simulink model "cic"  (Simulink 7.1)
settings: Solver=FixedStepDiscrete  StartTime=0.0  StopTime=400  RelTol=1e-3
PreLoadFcn:
  | topiirinit
InitFcn:
  | %% DSPBuilder Start
  | alt_dspbuilder_update_model(bdroot)
  | %% DSPBuilder End
libraries: allblocks_alteradspbuilder2 x17
settings Model: Creator=mjervis  LastModifiedBy=Bass
settings DataIOCC: SignalLoggingName=sigsOut
settings OptimizationCC: BooleanDataType=off  InlineInvariantSignals=on
settings DebuggingCC: SaveWithParameterizedLinksMsg=none  SignalResolutionControl=TryResolveAllWithWarning  SolverPrmCheckMsg=none  MultiTaskDSMMsg=warning  MultiTaskCondExecSysMsg=none
settings HardwareCC: TargetEndianess=LittleEndian  TargetHWDeviceType=MATLAB Host  ProdEqTarget=off
settings RTWCC: IncludeERTFirstTime=on
settings GRTTargetCC: TargetFcnLib=ansi_tfl_tmw.mat

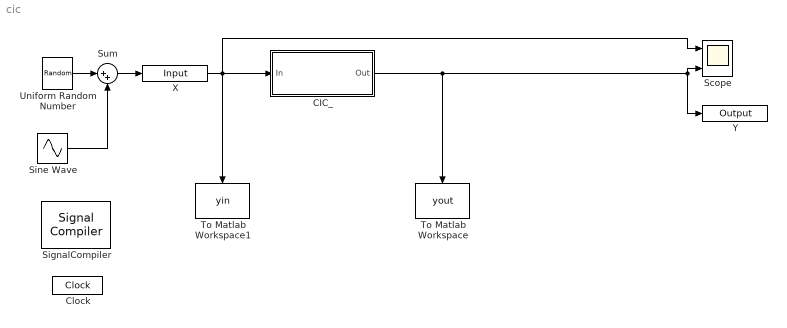
== system cic ==
  CIC_ : Subsystem
  Clock : allblocks_alteradspbuilder2/Clock  ClockPeriod=16  ClockPeriodUnit=ns  SampleTime=1  SimulationStartCycle=5  PhaseOffset=0  Reset=aclr  ResetType=Active Low  Export=off
  Scope : Scope  NumInputPorts=2
      settings: TimeRange=100  YMin=-0.1~-1000  YMax=0.4~1000
  SignalCompiler : allblocks_alteradspbuilder2/Signal Compiler  DeviceFamily=Cyclone  DeviceName=AUTO  EnableSignalTap=off  SignalTapDepth=128  UseBoardBlock=off  StpUseDefaultClock=on  StpClock=Clock  ExportDir=C:\Documents and Settings\Bass\My Documents\MATLAB
  Sine Wave : Sin  SineType=Sample based  TimeSource=Use external signal  Amplitude=1000  Frequency=0.25  Samples=5  SampleTime=0
  Sum : Sum  Inputs=|++  OutDataType=sfix(16)  OutScaling=2^0
  To Matlab Workspace : ToWorkspace  VariableName=yout  SampleTime=-1  SaveFormat=Array
      settings: Orientation=down
  To Matlab Workspace1 : ToWorkspace  VariableName=yin  SampleTime=-1  SaveFormat=Array
      settings: Orientation=down
  Uniform Random Number : UniformRandomNumber  Minimum=0  SampleTime=1
  X : allblocks_alteradspbuilder2/Input  iofile=C:\Documents and Settings\Bass\My Documents\MATLAB\MFC_Simul\CIC\tb_cic\cic_X.salt  BusType=Signed Integer  bwl=12  bwr=8  SpecifyClock=off  PORTTYPE=Input  externalType=Inferred  allowFloatingPointOverride=on  logOutputs=off
  Y : allblocks_alteradspbuilder2/Output  iofile=C:\Documents and Settings\Bass\My Documents\MATLAB\MFC_Simul\CIC\tb_cic\cic_Y.capture  BusType=Signed Integer  bwl=16  bwr=12  externalType=Inferred  PORTTYPE=Output  allowFloatingPointOverride=on  logOutputs=off
  wires:
  X/1 -> Scope/1, To Matlab Workspace1/1, CIC_/1(In)
  Sum/1 -> X/1
  Uniform Random Number/1 -> Sum/1
  Sine Wave/1 -> Sum/2
  CIC_/1(Out) -> To Matlab Workspace/1, Scope/2, Y/1

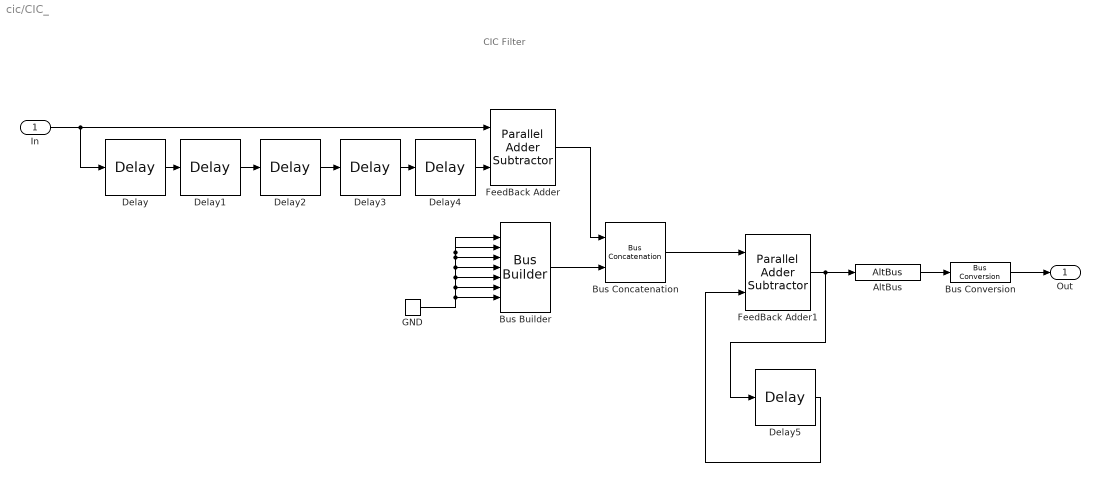
== system cic/CIC_ ==
  note: CIC Filter
  In : Inport  OutDataType=sfix(16)  OutScaling=2^0
  AltBus : allblocks_alteradspbuilder2/AltBus  BusType=Signed Integer  bwl=19  bwr=0  saturate=off  floatingPointInput=on  floatingPointOutput=on  logOutputs=off  logFile=C:\Documents and Settings\Bass\My Documents\MATLAB\MFC_Simul\CIC\tb_cic\cic_CIC%5F_AltBus.fixedpointlog
  Bus Builder : allblocks_alteradspbuilder2/Bus Builder  BusType=Signed Integer  bwl=7  bwr=1  pipeline_display=0
  Bus Concatenation : allblocks_alteradspbuilder2/Bus Concatenation  isSigned=off  awidth=12  bwidth=7  pipeline_display=0
  Bus Conversion : allblocks_alteradspbuilder2/Bus Conversion  BusType=Signed Integer  ibwl=19  ibwr=1  bwl=16  bwr=1  bitToConnectToOutputLSB=3  round=off  saturate=off  pipeline_display=0
  Delay : allblocks_alteradspbuilder2/Delay  pipeline=1  pipeline_display=1  ClockPhase=1  use_ena=off  use_sclr=off  allowFloatingPointOverride=on  logOutputs=off  logFile=C:\Documents and Settings\Bass\My Documents\MATLAB\MFC_Simul\CIC\tb_cic\cic_CIC%5F_Delay.fixedpointlog  use_init=off  reset_value=1
  Delay1 : allblocks_alteradspbuilder2/Delay  pipeline=1  pipeline_display=1  ClockPhase=1  use_ena=off  use_sclr=off  allowFloatingPointOverride=on  logOutputs=off  logFile=C:\Documents and Settings\Bass\My Documents\MATLAB\MFC_Simul\CIC\tb_cic\cic_CIC%5F_Delay1.fixedpointlog  use_init=off  reset_value=1
  Delay2 : allblocks_alteradspbuilder2/Delay  pipeline=1  pipeline_display=1  ClockPhase=1  use_ena=off  use_sclr=off  allowFloatingPointOverride=on  logOutputs=off  logFile=C:\Documents and Settings\Bass\My Documents\MATLAB\MFC_Simul\CIC\tb_cic\cic_CIC%5F_Delay2.fixedpointlog  use_init=off  reset_value=1
  Delay3 : allblocks_alteradspbuilder2/Delay  pipeline=1  pipeline_display=1  ClockPhase=1  use_ena=off  use_sclr=off  allowFloatingPointOverride=on  logOutputs=off  logFile=C:\Documents and Settings\Bass\My Documents\MATLAB\MFC_Simul\CIC\tb_cic\cic_CIC%5F_Delay3.fixedpointlog  use_init=off  reset_value=1
  Delay4 : allblocks_alteradspbuilder2/Delay  pipeline=1  pipeline_display=1  ClockPhase=1  use_ena=off  use_sclr=off  allowFloatingPointOverride=on  logOutputs=off  logFile=C:\Documents and Settings\Bass\My Documents\MATLAB\MFC_Simul\CIC\tb_cic\cic_CIC%5F_Delay4.fixedpointlog  use_init=off  reset_value=1
  Delay5 : allblocks_alteradspbuilder2/Delay  pipeline=1  pipeline_display=1  ClockPhase=1  use_ena=off  use_sclr=off  allowFloatingPointOverride=on  logOutputs=off  logFile=C:\Documents and Settings\Bass\My Documents\MATLAB\MFC_Simul\CIC\tb_cic\cic_CIC%5F_Delay5.fixedpointlog  use_init=off  reset_value=1
  FeedBack Adder : allblocks_alteradspbuilder2/Parallel Adder Subtractor  number_of_inputs=2  direction=+-  use_pipeline=on  pipeline_display=1  phase_selection=1  use_ena=off  use_aclr=off  allowFloatingPointOverride=on  logOutputs=off  logFile=C:\Documents and Settings\Bass\My Documents\MATLAB\MFC_Simul\CIC\tb_cic\cic_CIC%5F_FeedBack+Adder.fixedpointlog
  FeedBack Adder1 : allblocks_alteradspbuilder2/Parallel Adder Subtractor  number_of_inputs=2  direction=++  use_pipeline=on  pipeline_display=1  phase_selection=1  use_ena=off  use_aclr=off  allowFloatingPointOverride=on  logOutputs=off  logFile=C:\Documents and Settings\Bass\My Documents\MATLAB\MFC_Simul\CIC\tb_cic\cic_CIC%5F_FeedBack+Adder1.fixedpointlog
  GND : allblocks_alteradspbuilder2/GND  SpecifyClock=off
  Out : Outport  OutDataType=sfix(16)  OutScaling=2^0
  wires:
  In/1 -> FeedBack Adder/1, Delay/1
  Delay/1 -> Delay1/1
  Delay1/1 -> Delay2/1
  Delay2/1 -> Delay3/1
  Delay3/1 -> Delay4/1
  Delay4/1 -> FeedBack Adder/2
  Delay5/1 -> FeedBack Adder1/2
  FeedBack Adder1/1 -> Delay5/1, AltBus/1
  AltBus/1 -> Bus Conversion/1
  Bus Conversion/1 -> Out/1
  FeedBack Adder/1 -> Bus Concatenation/1
  Bus Concatenation/1 -> FeedBack Adder1/1
  Bus Builder/1 -> Bus Concatenation/2
  GND/1 -> Bus Builder/7, Bus Builder/1, Bus Builder/2, Bus Builder/3, Bus Builder/4, Bus Builder/5, Bus Builder/6
